simulink model "SingleMinima"  (R2016a)
settings: Solver=FixedStepAuto  StartTime=0.0  StopTime=10.0  RelTol=1e-3
undefined symbols (not defined in the file): const
settings Model: Creator=Josef  LastModifiedBy=Josef
settings GRTTargetCC: GeneratePreprocessorConditionals=Use local settings

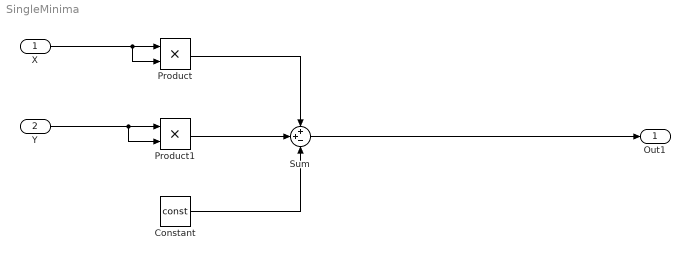
== system SingleMinima ==
  X : Inport
  Y : Inport  Port=2
  Constant : Constant  Value=const
  Product : Product
  Product1 : Product
  Sum : Sum  Inputs=++-
  Out1 : Outport
  wires:
  X/1 -> Product/2, Product/1
  Y/1 -> Product1/2, Product1/1
  Constant/1 -> Sum/3
  Product/1 -> Sum/1
  Product1/1 -> Sum/2
  Sum/1 -> Out1/1
